simulink model "atividade2_Simulacao"  (Simulink 7.1)
settings: Solver=ode45  StartTime=0.0  StopTime=10.0  RelTol=1e-3
settings Model: Creator=CARLOS BRUNO  LastModifiedBy=CARLOS BRUNO

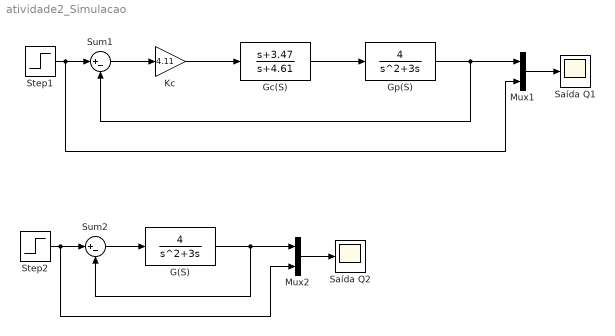
== system atividade2_Simulacao ==
  G(S) : TransferFcn  Numerator=[4]  Denominator="[1  3 0]"
  Gc(S) : TransferFcn  Numerator=[1 3.47]  Denominator=[1 4.61]
  Gp(S) : TransferFcn  Numerator=[4]  Denominator="[1  3 0]"
  Kc : Gain  Gain=4.11  ParameterDataType=sfix(16)  ParameterScaling=2^0  OutDataType=sfix(16)  OutScaling=2^0
  Mux1 : Mux  Inputs=2
  Mux2 : Mux  Inputs=2
  Saída Q1 : Scope
      settings: TimeRange=20  YMin=5.55112e-017  YMax=1
  Saída Q2 : Scope
      settings: TimeRange=20  YMin=5.55112e-017  YMax=1
  Step1 : Step  Time=0  SampleTime=0
  Step2 : Step  Time=0  SampleTime=0
  Sum1 : Sum  Inputs=|+-  OutDataType=sfix(16)  OutScaling=2^0
  Sum2 : Sum  Inputs=|+-  OutDataType=sfix(16)  OutScaling=2^0
  wires:
  Step1/1 -> Sum1/1, Mux1/2
  Mux1/1 -> Saída Q1/1
  Gp(S)/1 -> Mux1/1, Sum1/2
  Sum1/1 -> Kc/1
  Gc(S)/1 -> Gp(S)/1
  Kc/1 -> Gc(S)/1
  Step2/1 -> Sum2/1, Mux2/2
  Mux2/1 -> Saída Q2/1
  G(S)/1 -> Mux2/1, Sum2/2
  Sum2/1 -> G(S)/1
